simulink model "Controller_Exp"  (R2016a)
settings: Solver=ode4  StartTime=0.0  StopTime=Inf  FixedStep=Ts  RelTol=1e-3
undefined symbols (not defined in the file or in its folder): A_lpf_velocity, B1_lpf_velocity, B2_lpf_velocity, Calibration, commanded_u, GearOffsets, IMUTorsoOffsets, MedullaCommand, ResetDAQ, sample_time, TorsoCOMOffsets, Ts
libraries: xpcethercatlib x188, simulink x37, slrtlib x11, ControllerLibrary x2, dspswit3 x1
(part 3 of 4)

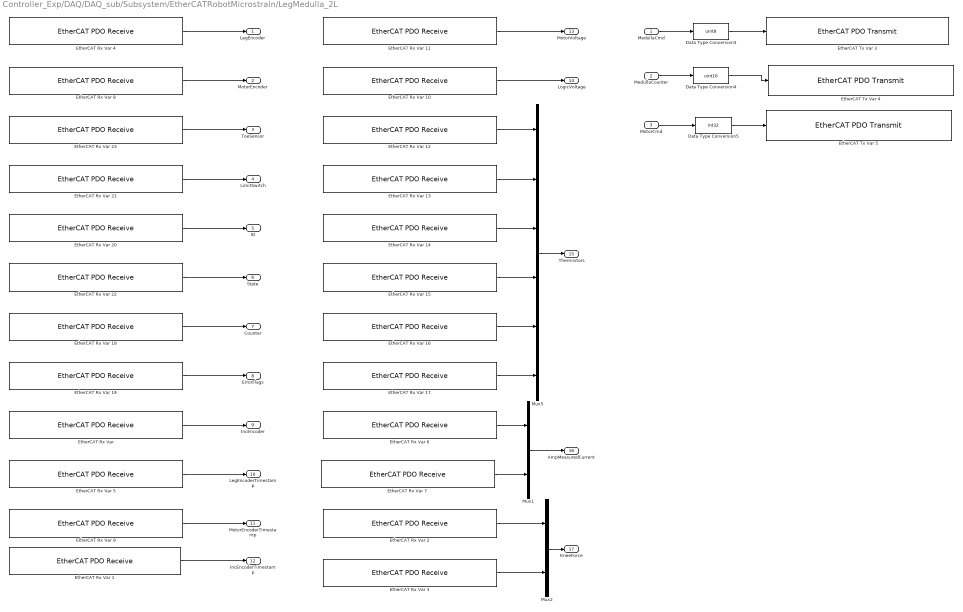
== system Controller_Exp/DAQ/DAQ_sub/Subsystem/EtherCATRobotMicrostrain/LegMedulla_2L ==
  MedullaCmd : Inport
  MedullaCounter : Inport  Port=2
  MotorCmd : Inport  Port=3
  Data Type Conversion3 : DataTypeConversion  OutDataTypeStr=uint8  RndMeth=Simplest
  Data Type Conversion4 : DataTypeConversion  OutDataTypeStr=uint16  RndMeth=Simplest
  Data Type Conversion5 : DataTypeConversion  OutDataTypeStr=int32  RndMeth=Simplest
  "EtherCAT Rx Var " : xpcethercatlib/EtherCAT PDO Receive  Priority=2  sig_name=Box 6 (ATRIAS 2.1 Leg (Medulla 1.5)).Incremental Encoder.Incremental Encoder  sig_offset=1624  sig_type=uint16  type_size=16  sig_dim=1  device_id=3  sample_time=0.001000
  EtherCAT Rx Var 1 : xpcethercatlib/EtherCAT PDO Receive  Priority=2  sig_name=Box 6 (ATRIAS 2.1 Leg (Medulla 1.5)).Incremental Encoder.Incremental Encoder Timestamp  sig_offset=1640  sig_type=uint16  type_size=16  sig_dim=1  device_id=3  sample_time=0.001000
  EtherCAT Rx Var 10 : xpcethercatlib/EtherCAT PDO Receive  Priority=2  sig_name=Box 6 (ATRIAS 2.1 Leg (Medulla 1.5)).Power.Logic Voltage  sig_offset=1672  sig_type=uint16  type_size=16  sig_dim=1  device_id=3  sample_time=0.001000
  EtherCAT Rx Var 11 : xpcethercatlib/EtherCAT PDO Receive  Priority=2  sig_name=Box 6 (ATRIAS 2.1 Leg (Medulla 1.5)).Power.Motor Voltage  sig_offset=1656  sig_type=uint16  type_size=16  sig_dim=1  device_id=3  sample_time=0.001000
  EtherCAT Rx Var 12 : xpcethercatlib/EtherCAT PDO Receive  Priority=2  sig_name=Box 6 (ATRIAS 2.1 Leg (Medulla 1.5)).Thermistors.Thermistor 0  sig_offset=1688  sig_type=uint16  type_size=16  sig_dim=1  device_id=3  sample_time=0.001000
  EtherCAT Rx Var 13 : xpcethercatlib/EtherCAT PDO Receive  Priority=2  sig_name=Box 6 (ATRIAS 2.1 Leg (Medulla 1.5)).Thermistors.Thermistor 1  sig_offset=1704  sig_type=uint16  type_size=16  sig_dim=1  device_id=3  sample_time=0.001000
  EtherCAT Rx Var 14 : xpcethercatlib/EtherCAT PDO Receive  Priority=2  sig_name=Box 6 (ATRIAS 2.1 Leg (Medulla 1.5)).Thermistors.Thermistor 2  sig_offset=1720  sig_type=uint16  type_size=16  sig_dim=1  device_id=3  sample_time=0.001000
  EtherCAT Rx Var 15 : xpcethercatlib/EtherCAT PDO Receive  Priority=2  sig_name=Box 6 (ATRIAS 2.1 Leg (Medulla 1.5)).Thermistors.Thermistor 3  sig_offset=1736  sig_type=uint16  type_size=16  sig_dim=1  device_id=3  sample_time=0.001000
  EtherCAT Rx Var 16 : xpcethercatlib/EtherCAT PDO Receive  Priority=2  sig_name=Box 6 (ATRIAS 2.1 Leg (Medulla 1.5)).Thermistors.Thermistor 4  sig_offset=1752  sig_type=uint16  type_size=16  sig_dim=1  device_id=3  sample_time=0.001000
  EtherCAT Rx Var 17 : xpcethercatlib/EtherCAT PDO Receive  Priority=2  sig_name=Box 6 (ATRIAS 2.1 Leg (Medulla 1.5)).Thermistors.Thermistor 5  sig_offset=1768  sig_type=uint16  type_size=16  sig_dim=1  device_id=3  sample_time=0.001000
  EtherCAT Rx Var 18 : xpcethercatlib/EtherCAT PDO Receive  Priority=2  sig_name=Box 6 (ATRIAS 2.1 Leg (Medulla 1.5)).uController Status.Counter  sig_offset=1488  sig_type=uint8  type_size=8  sig_dim=1  device_id=3  sample_time=0.001000
  EtherCAT Rx Var 19 : xpcethercatlib/EtherCAT PDO Receive  Priority=2  sig_name=Box 6 (ATRIAS 2.1 Leg (Medulla 1.5)).uController Status.Error Flags  sig_offset=1496  sig_type=uint8  type_size=8  sig_dim=1  device_id=3  sample_time=0.001000
  EtherCAT Rx Var 2 : xpcethercatlib/EtherCAT PDO Receive  Priority=2  sig_name=Box 6 (ATRIAS 2.1 Leg (Medulla 1.5)).Knee Force.Knee Force 1  sig_offset=1816  sig_type=uint16  type_size=16  sig_dim=1  device_id=3  sample_time=0.001000
  EtherCAT Rx Var 20 : xpcethercatlib/EtherCAT PDO Receive  Priority=2  sig_name=Box 6 (ATRIAS 2.1 Leg (Medulla 1.5)).uController Status.ID  sig_offset=1472  sig_type=uint8  type_size=8  sig_dim=1  device_id=3  sample_time=0.001000
  EtherCAT Rx Var 21 : xpcethercatlib/EtherCAT PDO Receive  Priority=2  sig_name=Box 6 (ATRIAS 2.1 Leg (Medulla 1.5)).uController Status.Limit Switch  sig_offset=1504  sig_type=uint8  type_size=8  sig_dim=1  device_id=3  sample_time=0.001000
  EtherCAT Rx Var 22 : xpcethercatlib/EtherCAT PDO Receive  Priority=2  sig_name=Box 6 (ATRIAS 2.1 Leg (Medulla 1.5)).uController Status.State  sig_offset=1480  sig_type=uint8  type_size=8  sig_dim=1  device_id=3  sample_time=0.001000
  EtherCAT Rx Var 23 : xpcethercatlib/EtherCAT PDO Receive  Priority=2  sig_name=Box 6 (ATRIAS 2.1 Leg (Medulla 1.5)).uController Status.Toe Sensor  sig_offset=1512  sig_type=uint16  type_size=16  sig_dim=1  device_id=3  sample_time=0.001000
  EtherCAT Rx Var 3 : xpcethercatlib/EtherCAT PDO Receive  Priority=2  sig_name=Box 6 (ATRIAS 2.1 Leg (Medulla 1.5)).Knee Force.Knee Force 2  sig_offset=1832  sig_type=uint16  type_size=16  sig_dim=1  device_id=3  sample_time=0.001000
  EtherCAT Rx Var 4 : xpcethercatlib/EtherCAT PDO Receive  Priority=2  sig_name=Box 6 (ATRIAS 2.1 Leg (Medulla 1.5)).Leg Encoder.Leg Encoder  sig_offset=1576  sig_type=uint32  type_size=32  sig_dim=1  device_id=3  sample_time=0.001000
  EtherCAT Rx Var 5 : xpcethercatlib/EtherCAT PDO Receive  Priority=2  sig_name=Box 6 (ATRIAS 2.1 Leg (Medulla 1.5)).Leg Encoder.Leg Encoder Timestamp  sig_offset=1608  sig_type=uint16  type_size=16  sig_dim=1  device_id=3  sample_time=0.001000
  EtherCAT Rx Var 6 : xpcethercatlib/EtherCAT PDO Receive  Priority=2  sig_name=Box 6 (ATRIAS 2.1 Leg (Medulla 1.5)).Measured Current.Amp 1 Measured Current  sig_offset=1784  sig_type=int16  type_size=16  sig_dim=1  device_id=3  sample_time=0.001000
  EtherCAT Rx Var 7 : xpcethercatlib/EtherCAT PDO Receive  Priority=2  sig_name=Box 6 (ATRIAS 2.1 Leg (Medulla 1.5)).Measured Current.Amp 2 Measured Current  sig_offset=1800  sig_type=int16  type_size=16  sig_dim=1  device_id=3  sample_time=0.001000
  EtherCAT Rx Var 8 : xpcethercatlib/EtherCAT PDO Receive  Priority=2  sig_name=Box 6 (ATRIAS 2.1 Leg (Medulla 1.5)).Motor Encoder.Motor Encoder  sig_offset=1528  sig_type=uint32  type_size=32  sig_dim=1  device_id=3  sample_time=0.001000
  EtherCAT Rx Var 9 : xpcethercatlib/EtherCAT PDO Receive  Priority=2  sig_name=Box 6 (ATRIAS 2.1 Leg (Medulla 1.5)).Motor Encoder.Motor Encoder Timestamp  sig_offset=1560  sig_type=uint16  type_size=16  sig_dim=1  device_id=3  sample_time=0.001000
  EtherCAT Tx Var 3 : xpcethercatlib/EtherCAT PDO Transmit   Priority=3  sig_name=Box 6 (ATRIAS 2.1 Leg (Medulla 1.5)).uControllerInput.Command  sig_offset=1472  sig_type=uint8  type_size=8  sig_dim=1  device_id=3  sample_time=0.001000
  EtherCAT Tx Var 4 : xpcethercatlib/EtherCAT PDO Transmit   Priority=3  sig_name=Box 6 (ATRIAS 2.1 Leg (Medulla 1.5)).uControllerInput.Counter  sig_offset=1480  sig_type=uint16  type_size=16  sig_dim=1  device_id=3  sample_time=0.001000
  EtherCAT Tx Var 5 : xpcethercatlib/EtherCAT PDO Transmit   Priority=3  sig_name=Box 6 (ATRIAS 2.1 Leg (Medulla 1.5)).uControllerInput.Motor Current  sig_offset=1496  sig_type=int32  type_size=32  sig_dim=1  device_id=3  sample_time=0.001000
  Mux1 : Mux  Inputs=2
  Mux2 : Mux  Inputs=2
  Mux5 : Mux  Inputs=6
  LegEncoder : Outport
  MotorEncoder : Outport  Port=2
  ToeSensor : Outport  Port=3
  LimitSwitch : Outport  Port=4
  ID : Outport  Port=5
  State : Outport  Port=6
  Counter : Outport  Port=7
  ErrorFlags : Outport  Port=8
  IncEncoder : Outport  Port=9
  LegEncoderTimestamp : Outport  Port=10
  MotorEncoderTimestamp : Outport  Port=11
  IncEncoderTimestamp : Outport  Port=12
  MotorVoltage : Outport  Port=13
  LogicVoltage : Outport  Port=14
  Thermistors : Outport  Port=15
  AmpMeasuredCurrent : Outport  Port=16
  KneeForce : Outport  Port=17
  wires:
  Mux2/1 -> KneeForce/1
  Mux1/1 -> AmpMeasuredCurrent/1
  Mux5/1 -> Thermistors/1
  MotorCmd/1 -> Data Type Conversion5/1
  MedullaCounter/1 -> Data Type Conversion4/1
  MedullaCmd/1 -> Data Type Conversion3/1
  EtherCAT Rx Var 23/1 -> ToeSensor/1
  EtherCAT Rx Var 22/1 -> State/1
  EtherCAT Rx Var 21/1 -> LimitSwitch/1
  EtherCAT Rx Var 20/1 -> ID/1
  EtherCAT Rx Var 19/1 -> ErrorFlags/1
  EtherCAT Rx Var 18/1 -> Counter/1
  EtherCAT Rx Var 17/1 -> Mux5/6
  EtherCAT Rx Var 16/1 -> Mux5/5
  EtherCAT Rx Var 15/1 -> Mux5/4
  EtherCAT Rx Var 14/1 -> Mux5/3
  EtherCAT Rx Var 13/1 -> Mux5/2
  EtherCAT Rx Var 12/1 -> Mux5/1
  EtherCAT Rx Var 11/1 -> MotorVoltage/1
  EtherCAT Rx Var 10/1 -> LogicVoltage/1
  EtherCAT Rx Var 9/1 -> MotorEncoderTimestamp/1
  EtherCAT Rx Var 8/1 -> MotorEncoder/1
  EtherCAT Rx Var 7/1 -> Mux1/2
  EtherCAT Rx Var 6/1 -> Mux1/1
  EtherCAT Rx Var 5/1 -> LegEncoderTimestamp/1
  EtherCAT Rx Var 4/1 -> LegEncoder/1
  EtherCAT Rx Var 3/1 -> Mux2/2
  EtherCAT Rx Var 2/1 -> Mux2/1
  EtherCAT Rx Var 1/1 -> IncEncoderTimestamp/1
  "EtherCAT Rx Var "/1 -> IncEncoder/1
  Data Type Conversion5/1 -> EtherCAT Tx Var 5/1
  Data Type Conversion4/1 -> EtherCAT Tx Var 4/1
  Data Type Conversion3/1 -> EtherCAT Tx Var 3/1

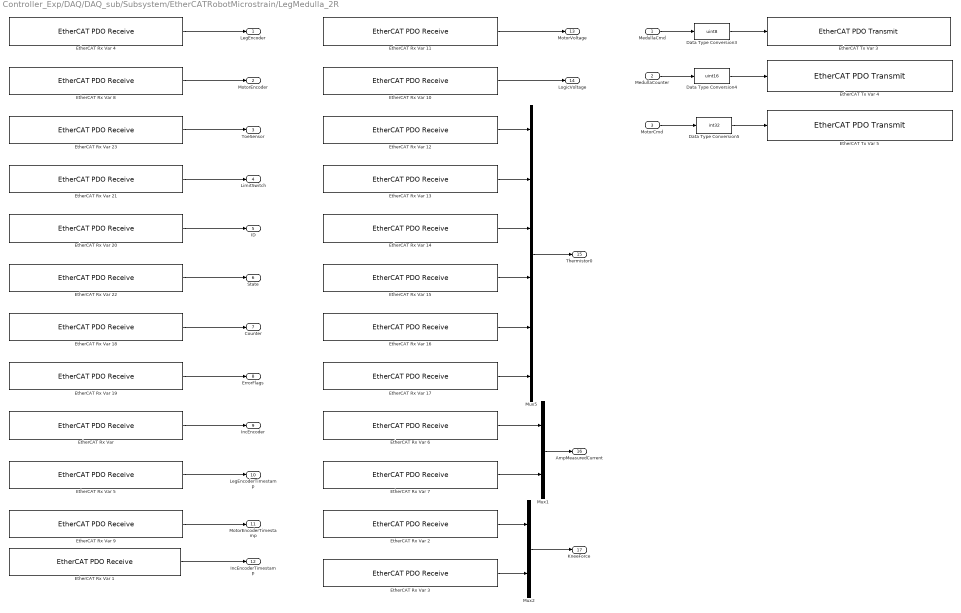
== system Controller_Exp/DAQ/DAQ_sub/Subsystem/EtherCATRobotMicrostrain/LegMedulla_2R ==
  MedullaCmd : Inport
  MedullaCounter : Inport  Port=2
  MotorCmd : Inport  Port=3
  Data Type Conversion3 : DataTypeConversion  OutDataTypeStr=uint8  RndMeth=Simplest
  Data Type Conversion4 : DataTypeConversion  OutDataTypeStr=uint16  RndMeth=Simplest
  Data Type Conversion5 : DataTypeConversion  OutDataTypeStr=int32  RndMeth=Simplest
  "EtherCAT Rx Var " : xpcethercatlib/EtherCAT PDO Receive  Priority=2  sig_name=Box 7 (ATRIAS 2.1 Leg (Medulla 1.5)).Incremental Encoder.Incremental Encoder  sig_offset=2000  sig_type=uint16  type_size=16  sig_dim=1  device_id=3  sample_time=0.001000
  EtherCAT Rx Var 1 : xpcethercatlib/EtherCAT PDO Receive  Priority=2  sig_name=Box 7 (ATRIAS 2.1 Leg (Medulla 1.5)).Incremental Encoder.Incremental Encoder Timestamp  sig_offset=2016  sig_type=uint16  type_size=16  sig_dim=1  device_id=3  sample_time=0.001000
  EtherCAT Rx Var 10 : xpcethercatlib/EtherCAT PDO Receive  Priority=2  sig_name=Box 7 (ATRIAS 2.1 Leg (Medulla 1.5)).Power.Logic Voltage  sig_offset=2048  sig_type=uint16  type_size=16  sig_dim=1  device_id=3  sample_time=0.001000
  EtherCAT Rx Var 11 : xpcethercatlib/EtherCAT PDO Receive  Priority=2  sig_name=Box 7 (ATRIAS 2.1 Leg (Medulla 1.5)).Power.Motor Voltage  sig_offset=2032  sig_type=uint16  type_size=16  sig_dim=1  device_id=3  sample_time=0.001000
  EtherCAT Rx Var 12 : xpcethercatlib/EtherCAT PDO Receive  Priority=2  sig_name=Box 7 (ATRIAS 2.1 Leg (Medulla 1.5)).Thermistors.Thermistor 0  sig_offset=2064  sig_type=uint16  type_size=16  sig_dim=1  device_id=3  sample_time=0.001000
  EtherCAT Rx Var 13 : xpcethercatlib/EtherCAT PDO Receive  Priority=2  sig_name=Box 7 (ATRIAS 2.1 Leg (Medulla 1.5)).Thermistors.Thermistor 1  sig_offset=2080  sig_type=uint16  type_size=16  sig_dim=1  device_id=3  sample_time=0.001000
  EtherCAT Rx Var 14 : xpcethercatlib/EtherCAT PDO Receive  Priority=2  sig_name=Box 7 (ATRIAS 2.1 Leg (Medulla 1.5)).Thermistors.Thermistor 2  sig_offset=2096  sig_type=uint16  type_size=16  sig_dim=1  device_id=3  sample_time=0.001000
  EtherCAT Rx Var 15 : xpcethercatlib/EtherCAT PDO Receive  Priority=2  sig_name=Box 7 (ATRIAS 2.1 Leg (Medulla 1.5)).Thermistors.Thermistor 3  sig_offset=2112  sig_type=uint16  type_size=16  sig_dim=1  device_id=3  sample_time=0.001000
  EtherCAT Rx Var 16 : xpcethercatlib/EtherCAT PDO Receive  Priority=2  sig_name=Box 7 (ATRIAS 2.1 Leg (Medulla 1.5)).Thermistors.Thermistor 4  sig_offset=2128  sig_type=uint16  type_size=16  sig_dim=1  device_id=3  sample_time=0.001000
  EtherCAT Rx Var 17 : xpcethercatlib/EtherCAT PDO Receive  Priority=2  sig_name=Box 7 (ATRIAS 2.1 Leg (Medulla 1.5)).Thermistors.Thermistor 5  sig_offset=2144  sig_type=uint16  type_size=16  sig_dim=1  device_id=3  sample_time=0.001000
  EtherCAT Rx Var 18 : xpcethercatlib/EtherCAT PDO Receive  Priority=2  sig_name=Box 7 (ATRIAS 2.1 Leg (Medulla 1.5)).uController Status.Counter  sig_offset=1864  sig_type=uint8  type_size=8  sig_dim=1  device_id=3  sample_time=0.001000
  EtherCAT Rx Var 19 : xpcethercatlib/EtherCAT PDO Receive  Priority=2  sig_name=Box 7 (ATRIAS 2.1 Leg (Medulla 1.5)).uController Status.Error Flags  sig_offset=1872  sig_type=uint8  type_size=8  sig_dim=1  device_id=3  sample_time=0.001000
  EtherCAT Rx Var 2 : xpcethercatlib/EtherCAT PDO Receive  Priority=2  sig_name=Box 7 (ATRIAS 2.1 Leg (Medulla 1.5)).Knee Force.Knee Force 1  sig_offset=2192  sig_type=uint16  type_size=16  sig_dim=1  device_id=3  sample_time=0.001000
  EtherCAT Rx Var 20 : xpcethercatlib/EtherCAT PDO Receive  Priority=2  sig_name=Box 7 (ATRIAS 2.1 Leg (Medulla 1.5)).uController Status.ID  sig_offset=1848  sig_type=uint8  type_size=8  sig_dim=1  device_id=3  sample_time=0.001000
  EtherCAT Rx Var 21 : xpcethercatlib/EtherCAT PDO Receive  Priority=2  sig_name=Box 7 (ATRIAS 2.1 Leg (Medulla 1.5)).uController Status.Limit Switch  sig_offset=1880  sig_type=uint8  type_size=8  sig_dim=1  device_id=3  sample_time=0.001000
  EtherCAT Rx Var 22 : xpcethercatlib/EtherCAT PDO Receive  Priority=2  sig_name=Box 7 (ATRIAS 2.1 Leg (Medulla 1.5)).uController Status.State  sig_offset=1856  sig_type=uint8  type_size=8  sig_dim=1  device_id=3  sample_time=0.001000
  EtherCAT Rx Var 23 : xpcethercatlib/EtherCAT PDO Receive  Priority=2  sig_name=Box 7 (ATRIAS 2.1 Leg (Medulla 1.5)).uController Status.Toe Sensor  sig_offset=1888  sig_type=uint16  type_size=16  sig_dim=1  device_id=3  sample_time=0.001000
  EtherCAT Rx Var 3 : xpcethercatlib/EtherCAT PDO Receive  Priority=2  sig_name=Box 7 (ATRIAS 2.1 Leg (Medulla 1.5)).Knee Force.Knee Force 2  sig_offset=2208  sig_type=uint16  type_size=16  sig_dim=1  device_id=3  sample_time=0.001000
  EtherCAT Rx Var 4 : xpcethercatlib/EtherCAT PDO Receive  Priority=2  sig_name=Box 7 (ATRIAS 2.1 Leg (Medulla 1.5)).Leg Encoder.Leg Encoder  sig_offset=1952  sig_type=uint32  type_size=32  sig_dim=1  device_id=3  sample_time=0.001000
  EtherCAT Rx Var 5 : xpcethercatlib/EtherCAT PDO Receive  Priority=2  sig_name=Box 7 (ATRIAS 2.1 Leg (Medulla 1.5)).Leg Encoder.Leg Encoder Timestamp  sig_offset=1984  sig_type=uint16  type_size=16  sig_dim=1  device_id=3  sample_time=0.001000
  EtherCAT Rx Var 6 : xpcethercatlib/EtherCAT PDO Receive  Priority=2  sig_name=Box 7 (ATRIAS 2.1 Leg (Medulla 1.5)).Measured Current.Amp 1 Measured Current  sig_offset=2160  sig_type=int16  type_size=16  sig_dim=1  device_id=3  sample_time=0.001000
  EtherCAT Rx Var 7 : xpcethercatlib/EtherCAT PDO Receive  Priority=2  sig_name=Box 7 (ATRIAS 2.1 Leg (Medulla 1.5)).Measured Current.Amp 2 Measured Current  sig_offset=2176  sig_type=int16  type_size=16  sig_dim=1  device_id=3  sample_time=0.001000
  EtherCAT Rx Var 8 : xpcethercatlib/EtherCAT PDO Receive  Priority=2  sig_name=Box 7 (ATRIAS 2.1 Leg (Medulla 1.5)).Motor Encoder.Motor Encoder  sig_offset=1904  sig_type=uint32  type_size=32  sig_dim=1  device_id=3  sample_time=0.001000
  EtherCAT Rx Var 9 : xpcethercatlib/EtherCAT PDO Receive  Priority=2  sig_name=Box 7 (ATRIAS 2.1 Leg (Medulla 1.5)).Motor Encoder.Motor Encoder Timestamp  sig_offset=1936  sig_type=uint16  type_size=16  sig_dim=1  device_id=3  sample_time=0.001000
  EtherCAT Tx Var 3 : xpcethercatlib/EtherCAT PDO Transmit   Priority=3  sig_name=Box 7 (ATRIAS 2.1 Leg (Medulla 1.5)).uControllerInput.Command  sig_offset=1848  sig_type=uint8  type_size=8  sig_dim=1  device_id=3  sample_time=0.001000
  EtherCAT Tx Var 4 : xpcethercatlib/EtherCAT PDO Transmit   Priority=3  sig_name=Box 7 (ATRIAS 2.1 Leg (Medulla 1.5)).uControllerInput.Counter  sig_offset=1856  sig_type=uint16  type_size=16  sig_dim=1  device_id=3  sample_time=0.001000
  EtherCAT Tx Var 5 : xpcethercatlib/EtherCAT PDO Transmit   Priority=3  sig_name=Box 7 (ATRIAS 2.1 Leg (Medulla 1.5)).uControllerInput.Motor Current  sig_offset=1872  sig_type=int32  type_size=32  sig_dim=1  device_id=3  sample_time=0.001000
  Mux1 : Mux  Inputs=2
  Mux2 : Mux  Inputs=2
  Mux5 : Mux  Inputs=6
  LegEncoder : Outport
  MotorEncoder : Outport  Port=2
  ToeSensor : Outport  Port=3
  LimitSwitch : Outport  Port=4
  ID : Outport  Port=5
  State : Outport  Port=6
  Counter : Outport  Port=7
  ErrorFlags : Outport  Port=8
  IncEncoder : Outport  Port=9
  LegEncoderTimestamp : Outport  Port=10
  MotorEncoderTimestamp : Outport  Port=11
  IncEncoderTimestamp : Outport  Port=12
  MotorVoltage : Outport  Port=13
  LogicVoltage : Outport  Port=14
  Thermistor0 : Outport  Port=15
  AmpMeasuredCurrent : Outport  Port=16
  KneeForce : Outport  Port=17
  wires:
  Mux2/1 -> KneeForce/1
  Mux1/1 -> AmpMeasuredCurrent/1
  Mux5/1 -> Thermistor0/1
  MotorCmd/1 -> Data Type Conversion5/1
  MedullaCounter/1 -> Data Type Conversion4/1
  MedullaCmd/1 -> Data Type Conversion3/1
  EtherCAT Rx Var 23/1 -> ToeSensor/1
  EtherCAT Rx Var 22/1 -> State/1
  EtherCAT Rx Var 21/1 -> LimitSwitch/1
  EtherCAT Rx Var 20/1 -> ID/1
  EtherCAT Rx Var 19/1 -> ErrorFlags/1
  EtherCAT Rx Var 18/1 -> Counter/1
  EtherCAT Rx Var 17/1 -> Mux5/6
  EtherCAT Rx Var 16/1 -> Mux5/5
  EtherCAT Rx Var 15/1 -> Mux5/4
  EtherCAT Rx Var 14/1 -> Mux5/3
  EtherCAT Rx Var 13/1 -> Mux5/2
  EtherCAT Rx Var 12/1 -> Mux5/1
  EtherCAT Rx Var 11/1 -> MotorVoltage/1
  EtherCAT Rx Var 10/1 -> LogicVoltage/1
  EtherCAT Rx Var 9/1 -> MotorEncoderTimestamp/1
  EtherCAT Rx Var 8/1 -> MotorEncoder/1
  EtherCAT Rx Var 7/1 -> Mux1/2
  EtherCAT Rx Var 6/1 -> Mux1/1
  EtherCAT Rx Var 5/1 -> LegEncoderTimestamp/1
  EtherCAT Rx Var 4/1 -> LegEncoder/1
  EtherCAT Rx Var 3/1 -> Mux2/2
  EtherCAT Rx Var 2/1 -> Mux2/1
  EtherCAT Rx Var 1/1 -> IncEncoderTimestamp/1
  "EtherCAT Rx Var "/1 -> IncEncoder/1
  Data Type Conversion5/1 -> EtherCAT Tx Var 5/1
  Data Type Conversion4/1 -> EtherCAT Tx Var 4/1
  Data Type Conversion3/1 -> EtherCAT Tx Var 3/1

== system Controller_Exp/DAQ/DAQ_sub/Subsystem/EncoderFilters/Filter/Velocity Filter ==
  q : Inport
  Delay : Delay  DelayLength=1
  Delay1 : Delay
  Delay2 : Delay  DelayLength=3
  Delay3 : Delay  DelayLength=4
  Delay4 : Delay  DelayLength=5
  Delay5 : Delay  DelayLength=6
  Delay6 : Delay  DelayLength=7
  Delay7 : Delay  DelayLength=8
  Delay8 : Delay  DelayLength=9
  Median Filter : MATLAB Function  TreatAsAtomicUnit=on
  OSU_filter : Subsystem
  Vector Concatenate : Concatenate  NumInputs=9  Mode=Multidimensional array  ConcatenateDimension=2
  dq_out : Outport
  dq_original : Outport  Port=2
  wires:
  Median Filter/1(dq_out) -> dq_out/1
  q/1 -> OSU_filter/1(q)
  Vector Concatenate/1 -> Median Filter/2(dq_past)
  Delay/1 -> Vector Concatenate/1
  Delay1/1 -> Vector Concatenate/2
  Delay2/1 -> Vector Concatenate/3
  Delay3/1 -> Vector Concatenate/4
  Delay4/1 -> Vector Concatenate/5
  Delay5/1 -> Vector Concatenate/6
  Delay6/1 -> Vector Concatenate/7
  Delay7/1 -> Vector Concatenate/8
  Delay8/1 -> Vector Concatenate/9
  OSU_filter/1(dq) -> Median Filter/1(dq), Delay8/1, Delay7/1, Delay6/1, Delay5/1, Delay4/1, Delay3/1, Delay2/1, Delay1/1, Delay/1, dq_original/1

== system Controller_Exp/DAQ/DAQ_sub/Subsystem/EncoderFilters1/CheckAndFilterEncoder/Velocity Filter ==
  In1 : Inport
  Logic Filter : MATLAB Function  TreatAsAtomicUnit=on
  OSU_filter : Subsystem
  Unit Delay1 : UnitDelay  SampleTime=-1
  Unit Delay2 : UnitDelay  SampleTime=-1
  Out1 : Outport
  Out2 : Outport  Port=2
  wires:
  Logic Filter/1(dq_out) -> Out1/1
  OSU_filter/1(dq) -> Logic Filter/1(dq), Unit Delay2/1, Out2/1
  In1/1 -> OSU_filter/1(q)
  Unit Delay2/1 -> Logic Filter/2(dq_prev)
  Logic Filter/2(dq_good) -> Unit Delay1/1
  Unit Delay1/1 -> Logic Filter/3(dq_good_prev)

== system Controller_Exp/DAQ/DAQ_sub/Subsystem/EtherCATRobotMicrostrain/LegElmo_1L/EtherCATSubsystem ==
  TargetTorque : Inport
  ControlWord : Inport  Port=2
  ModeOfOperation : Inport  Port=3
  EtherCAT PDO Receive : xpcethercatlib/EtherCAT PDO Receive  Priority=2  sig_name=Box 3 (Elmo Drive).Inputs.Torque actual value  sig_offset=3024  sig_type=int16  type_size=16  sig_dim=1  device_id=3  sample_time=0.001000
  EtherCAT PDO Receive1 : xpcethercatlib/EtherCAT PDO Receive  Priority=2  sig_name=Box 3 (Elmo Drive).Inputs.Position actual value  sig_offset=2992  sig_type=int32  type_size=32  sig_dim=1  device_id=3  sample_time=0.001000
  EtherCAT PDO Receive2 : xpcethercatlib/EtherCAT PDO Receive  Priority=2  sig_name=Box 3 (Elmo Drive).Inputs.Mode of operation display  sig_offset=3056  sig_type=int8  type_size=8  sig_dim=1  device_id=3  sample_time=0.001000
  EtherCAT PDO Receive5 : xpcethercatlib/EtherCAT PDO Receive  Priority=2  sig_name=Box 3 (Elmo Drive).Inputs.Status word  sig_offset=3040  sig_type=uint16  type_size=16  sig_dim=1  device_id=3  sample_time=0.001000
  EtherCAT PDO Transmit : xpcethercatlib/EtherCAT PDO Transmit   Priority=3  sig_name=Box 3 (Elmo Drive).Outputs.Target Torque  sig_offset=2992  sig_type=int16  type_size=16  sig_dim=1  device_id=3  sample_time=0.001000
  EtherCAT PDO Transmit1 : xpcethercatlib/EtherCAT PDO Transmit   Priority=3  sig_name=Box 3 (Elmo Drive).Outputs.Control word  sig_offset=3008  sig_type=uint16  type_size=16  sig_dim=1  device_id=3  sample_time=0.001000
  EtherCAT PDO Transmit2 : xpcethercatlib/EtherCAT PDO Transmit   Priority=3  sig_name=Box 3 (Elmo Drive).Outputs.Mode of operation  sig_offset=3024  sig_type=int8  type_size=8  sig_dim=1  device_id=3  sample_time=0.001000
  TorqueActual : Outport
  ActualPosition : Outport  Port=2
  ModeOfOperationDisplay : Outport  Port=3
  StatusWord : Outport  Port=4
  wires:
  EtherCAT PDO Receive5/1 -> StatusWord/1
  TargetTorque/1 -> EtherCAT PDO Transmit/1
  EtherCAT PDO Receive2/1 -> ModeOfOperationDisplay/1
  ModeOfOperation/1 -> EtherCAT PDO Transmit2/1
  ControlWord/1 -> EtherCAT PDO Transmit1/1
  EtherCAT PDO Receive1/1 -> ActualPosition/1
  EtherCAT PDO Receive/1 -> TorqueActual/1

== system Controller_Exp/DAQ/DAQ_sub/Subsystem/EtherCATRobotMicrostrain/LegElmo_1L/Subsystem ==
  ActualValue : Inport
  MaxRatedCurrent : Inport  Port=2
  Data Type Conversion6 : DataTypeConversion  OutDataTypeStr=int16
  Fcn : Fcn  Expr=u(1)*1000/u(2)
  Vector Concatenate : Concatenate
  ScaledValue : Outport
  wires:
  Fcn/1 -> Data Type Conversion6/1
  Data Type Conversion6/1 -> ScaledValue/1
  MaxRatedCurrent/1 -> Vector Concatenate/2
  Vector Concatenate/1 -> Fcn/1
  ActualValue/1 -> Vector Concatenate/1

== system Controller_Exp/DAQ/DAQ_sub/Subsystem/EtherCATRobotMicrostrain/LegElmo_1L/Subsystem1 ==
  ControlWordIndex : Inport
  EnableControlWord : Subsystem
  FaultReset : Subsystem
  Merge : Merge  Inputs=4
  NothingControlWord : Subsystem
  ShutdownControlWord : Subsystem
  Switch Case : SwitchCase  CaseConditions={1,2,3}
  ControlWord : Outport
  wires:
  FaultReset/1(ControlWord) -> Merge/3
  Switch Case/3 -> FaultReset/Action
  EnableControlWord/1(ControlWord) -> Merge/2
  ControlWordIndex/1 -> Switch Case/1
  Switch Case/2 -> EnableControlWord/Action
  Switch Case/4 -> NothingControlWord/Action
  ShutdownControlWord/1(ControlWord) -> Merge/1
  Switch Case/1 -> ShutdownControlWord/Action
  Merge/1 -> ControlWord/1
  NothingControlWord/1(ControlWord) -> Merge/4

== system Controller_Exp/DAQ/DAQ_sub/Subsystem/EtherCATRobotMicrostrain/LegElmo_1L/Subsystem2 ==
  StatusWord : Inport
  Bitwise Operator : simulink/Logic and Bit Operations/Bitwise Operator  logicop=AND  UseBitMask=on  BitMask=bin2dec('0000000001001111')  BitMaskRealWorld=Stored Integer
  Compare To Constant : simulink/Logic and Bit Operations/Compare To Constant  relop===  const=bin2dec('0000000001000000')  OutDataTypeStr=boolean
  SwitchOnDisabledMode : Outport
  wires:
  Bitwise Operator/1 -> Compare To Constant/1
  Compare To Constant/1 -> SwitchOnDisabledMode/1
  StatusWord/1 -> Bitwise Operator/1

== system Controller_Exp/DAQ/DAQ_sub/Subsystem/EtherCATRobotMicrostrain/LegElmo_1L/Subsystem3 ==
  StatusWord : Inport
  Bitwise Operator : simulink/Logic and Bit Operations/Bitwise Operator  logicop=AND  UseBitMask=on  BitMask=bin2dec('0000000001101111')  BitMaskRealWorld=Stored Integer
  Compare To Constant : simulink/Logic and Bit Operations/Compare To Constant  relop===  const=bin2dec('0000000000100111')  OutDataTypeStr=boolean
  EnabledMode : Outport
  wires:
  Bitwise Operator/1 -> Compare To Constant/1
  Compare To Constant/1 -> EnabledMode/1
  StatusWord/1 -> Bitwise Operator/1

== system Controller_Exp/DAQ/DAQ_sub/Subsystem/EtherCATRobotMicrostrain/LegElmo_1L/Subsystem4 ==
  StatusWord : Inport
  Bitwise Operator : simulink/Logic and Bit Operations/Bitwise Operator  logicop=AND  UseBitMask=on  BitMask=bin2dec('0000000001101111')  BitMaskRealWorld=Stored Integer
  Compare To Constant : simulink/Logic and Bit Operations/Compare To Constant  relop===  const=bin2dec('0000000000100001')  OutDataTypeStr=boolean
  ReadyToSwitchOnMode : Outport
  wires:
  Bitwise Operator/1 -> Compare To Constant/1
  Compare To Constant/1 -> ReadyToSwitchOnMode/1
  StatusWord/1 -> Bitwise Operator/1

== system Controller_Exp/DAQ/DAQ_sub/Subsystem/EtherCATRobotMicrostrain/LegElmo_1L/Subsystem5 ==
  StatusWord : Inport
  Bitwise Operator : simulink/Logic and Bit Operations/Bitwise Operator  logicop=AND  UseBitMask=on  BitMask=bin2dec('0000000000001000')  BitMaskRealWorld=Stored Integer
  Compare To Constant : simulink/Logic and Bit Operations/Compare To Constant  relop===  const=bin2dec('0000000000001000')  OutDataTypeStr=boolean
  FaultMode : Outport
  wires:
  Bitwise Operator/1 -> Compare To Constant/1
  Compare To Constant/1 -> FaultMode/1
  StatusWord/1 -> Bitwise Operator/1

== system Controller_Exp/DAQ/DAQ_sub/Subsystem/EtherCATRobotMicrostrain/LegElmo_1L/Subsystem6 ==
  ScaledValue : Inport
  MaxRatedCurrent : Inport  Port=2
  Fcn : Fcn  Expr=u(1)*u(2)/1000
  Vector Concatenate : Concatenate
  ActualValue : Outport
  wires:
  Fcn/1 -> ActualValue/1
  MaxRatedCurrent/1 -> Vector Concatenate/2
  Vector Concatenate/1 -> Fcn/1
  ScaledValue/1 -> Vector Concatenate/1

== system Controller_Exp/DAQ/DAQ_sub/Subsystem/EtherCATRobotMicrostrain/LegElmo_1R/EtherCATSubsystem ==
  TargetTorque : Inport
  ControlWord : Inport  Port=2
  ModeOfOperation : Inport  Port=3
  EtherCAT PDO Receive : xpcethercatlib/EtherCAT PDO Receive  Priority=2  sig_name=Box 10 (Elmo Drive).Inputs.Torque actual value  sig_offset=3184  sig_type=int16  type_size=16  sig_dim=1  device_id=3  sample_time=0.001000
  EtherCAT PDO Receive1 : xpcethercatlib/EtherCAT PDO Receive  Priority=2  sig_name=Box 10 (Elmo Drive).Inputs.Position actual value  sig_offset=3152  sig_type=int32  type_size=32  sig_dim=1  device_id=3  sample_time=0.001000
  EtherCAT PDO Receive2 : xpcethercatlib/EtherCAT PDO Receive  Priority=2  sig_name=Box 10 (Elmo Drive).Inputs.Mode of operation display  sig_offset=3216  sig_type=int8  type_size=8  sig_dim=1  device_id=3  sample_time=0.001000
  EtherCAT PDO Receive5 : xpcethercatlib/EtherCAT PDO Receive  Priority=2  sig_name=Box 10 (Elmo Drive).Inputs.Status word  sig_offset=3200  sig_type=uint16  type_size=16  sig_dim=1  device_id=3  sample_time=0.001000
  EtherCAT PDO Transmit : xpcethercatlib/EtherCAT PDO Transmit   Priority=3  sig_name=Box 10 (Elmo Drive).Outputs.Target Torque  sig_offset=3152  sig_type=int16  type_size=16  sig_dim=1  device_id=3  sample_time=0.001000
  EtherCAT PDO Transmit1 : xpcethercatlib/EtherCAT PDO Transmit   Priority=3  sig_name=Box 10 (Elmo Drive).Outputs.Control word  sig_offset=3168  sig_type=uint16  type_size=16  sig_dim=1  device_id=3  sample_time=0.001000
  EtherCAT PDO Transmit2 : xpcethercatlib/EtherCAT PDO Transmit   Priority=3  sig_name=Box 10 (Elmo Drive).Outputs.Mode of operation  sig_offset=3184  sig_type=int8  type_size=8  sig_dim=1  device_id=3  sample_time=0.001000
  TorqueActual : Outport
  ActualPosition : Outport  Port=2
  ModeOfOperationDisplay : Outport  Port=3
  StatusWord : Outport  Port=4
  wires:
  EtherCAT PDO Receive5/1 -> StatusWord/1
  TargetTorque/1 -> EtherCAT PDO Transmit/1
  EtherCAT PDO Receive2/1 -> ModeOfOperationDisplay/1
  ModeOfOperation/1 -> EtherCAT PDO Transmit2/1
  ControlWord/1 -> EtherCAT PDO Transmit1/1
  EtherCAT PDO Receive1/1 -> ActualPosition/1
  EtherCAT PDO Receive/1 -> TorqueActual/1

== system Controller_Exp/DAQ/DAQ_sub/Subsystem/EtherCATRobotMicrostrain/LegElmo_1R/Subsystem ==
  ActualValue : Inport
  MaxRatedCurrent : Inport  Port=2
  Data Type Conversion6 : DataTypeConversion  OutDataTypeStr=int16
  Fcn : Fcn  Expr=u(1)*1000/u(2)
  Vector Concatenate : Concatenate
  ScaledValue : Outport
  wires:
  Fcn/1 -> Data Type Conversion6/1
  Data Type Conversion6/1 -> ScaledValue/1
  MaxRatedCurrent/1 -> Vector Concatenate/2
  Vector Concatenate/1 -> Fcn/1
  ActualValue/1 -> Vector Concatenate/1

== system Controller_Exp/DAQ/DAQ_sub/Subsystem/EtherCATRobotMicrostrain/LegElmo_1R/Subsystem1 ==
  ControlWordIndex : Inport
  EnableControlWord : Subsystem
  FaultReset : Subsystem
  Merge : Merge  Inputs=4
  NothingControlWord : Subsystem
  ShutdownControlWord : Subsystem
  Switch Case : SwitchCase  CaseConditions={1,2,3}
  ControlWord : Outport
  wires:
  FaultReset/1(ControlWord) -> Merge/3
  Switch Case/3 -> FaultReset/Action
  EnableControlWord/1(ControlWord) -> Merge/2
  ControlWordIndex/1 -> Switch Case/1
  Switch Case/2 -> EnableControlWord/Action
  Switch Case/4 -> NothingControlWord/Action
  ShutdownControlWord/1(ControlWord) -> Merge/1
  Switch Case/1 -> ShutdownControlWord/Action
  Merge/1 -> ControlWord/1
  NothingControlWord/1(ControlWord) -> Merge/4

== system Controller_Exp/DAQ/DAQ_sub/Subsystem/EtherCATRobotMicrostrain/LegElmo_1R/Subsystem2 ==
  StatusWord : Inport
  Bitwise Operator : simulink/Logic and Bit Operations/Bitwise Operator  logicop=AND  UseBitMask=on  BitMask=bin2dec('0000000001001111')  BitMaskRealWorld=Stored Integer
  Compare To Constant : simulink/Logic and Bit Operations/Compare To Constant  relop===  const=bin2dec('0000000001000000')  OutDataTypeStr=boolean
  SwitchOnDisabledMode : Outport
  wires:
  Bitwise Operator/1 -> Compare To Constant/1
  Compare To Constant/1 -> SwitchOnDisabledMode/1
  StatusWord/1 -> Bitwise Operator/1

== system Controller_Exp/DAQ/DAQ_sub/Subsystem/EtherCATRobotMicrostrain/LegElmo_1R/Subsystem3 ==
  StatusWord : Inport
  Bitwise Operator : simulink/Logic and Bit Operations/Bitwise Operator  logicop=AND  UseBitMask=on  BitMask=bin2dec('0000000001101111')  BitMaskRealWorld=Stored Integer
  Compare To Constant : simulink/Logic and Bit Operations/Compare To Constant  relop===  const=bin2dec('0000000000100111')  OutDataTypeStr=boolean
  EnabledMode : Outport
  wires:
  Bitwise Operator/1 -> Compare To Constant/1
  Compare To Constant/1 -> EnabledMode/1
  StatusWord/1 -> Bitwise Operator/1

== system Controller_Exp/DAQ/DAQ_sub/Subsystem/EtherCATRobotMicrostrain/LegElmo_1R/Subsystem4 ==
  StatusWord : Inport
  Bitwise Operator : simulink/Logic and Bit Operations/Bitwise Operator  logicop=AND  UseBitMask=on  BitMask=bin2dec('0000000001101111')  BitMaskRealWorld=Stored Integer
  Compare To Constant : simulink/Logic and Bit Operations/Compare To Constant  relop===  const=bin2dec('0000000000100001')  OutDataTypeStr=boolean
  ReadyToSwitchOnMode : Outport
  wires:
  Bitwise Operator/1 -> Compare To Constant/1
  Compare To Constant/1 -> ReadyToSwitchOnMode/1
  StatusWord/1 -> Bitwise Operator/1

== system Controller_Exp/DAQ/DAQ_sub/Subsystem/EtherCATRobotMicrostrain/LegElmo_1R/Subsystem5 ==
  StatusWord : Inport
  Bitwise Operator : simulink/Logic and Bit Operations/Bitwise Operator  logicop=AND  UseBitMask=on  BitMask=bin2dec('0000000000001000')  BitMaskRealWorld=Stored Integer
  Compare To Constant : simulink/Logic and Bit Operations/Compare To Constant  relop===  const=bin2dec('0000000000001000')  OutDataTypeStr=boolean
  FaultMode : Outport
  wires:
  Bitwise Operator/1 -> Compare To Constant/1
  Compare To Constant/1 -> FaultMode/1
  StatusWord/1 -> Bitwise Operator/1

== system Controller_Exp/DAQ/DAQ_sub/Subsystem/EtherCATRobotMicrostrain/LegElmo_1R/Subsystem6 ==
  ScaledValue : Inport
  MaxRatedCurrent : Inport  Port=2
  Fcn : Fcn  Expr=u(1)*u(2)/1000
  Vector Concatenate : Concatenate
  ActualValue : Outport
  wires:
  Fcn/1 -> ActualValue/1
  MaxRatedCurrent/1 -> Vector Concatenate/2
  Vector Concatenate/1 -> Fcn/1
  ScaledValue/1 -> Vector Concatenate/1

== system Controller_Exp/DAQ/DAQ_sub/Subsystem/EtherCATRobotMicrostrain/LegElmo_2L/EtherCATSubsystem ==
  TargetTorque : Inport
  ControlWord : Inport  Port=2
  ModeOfOperation : Inport  Port=3
  EtherCAT PDO Receive : xpcethercatlib/EtherCAT PDO Receive  Priority=2  sig_name=Box 2 (Elmo Drive).Inputs.Torque actual value  sig_offset=2944  sig_type=int16  type_size=16  sig_dim=1  device_id=3  sample_time=0.001000
  EtherCAT PDO Receive1 : xpcethercatlib/EtherCAT PDO Receive  Priority=2  sig_name=Box 2 (Elmo Drive).Inputs.Position actual value  sig_offset=2912  sig_type=int32  type_size=32  sig_dim=1  device_id=3  sample_time=0.001000
  EtherCAT PDO Receive2 : xpcethercatlib/EtherCAT PDO Receive  Priority=2  sig_name=Box 2 (Elmo Drive).Inputs.Mode of operation display  sig_offset=2976  sig_type=int8  type_size=8  sig_dim=1  device_id=3  sample_time=0.001000
  EtherCAT PDO Receive5 : xpcethercatlib/EtherCAT PDO Receive  Priority=2  sig_name=Box 2 (Elmo Drive).Inputs.Status word  sig_offset=2960  sig_type=uint16  type_size=16  sig_dim=1  device_id=3  sample_time=0.001000
  EtherCAT PDO Transmit : xpcethercatlib/EtherCAT PDO Transmit   Priority=3  sig_name=Box 2 (Elmo Drive).Outputs.Target Torque  sig_offset=2912  sig_type=int16  type_size=16  sig_dim=1  device_id=3  sample_time=0.001000
  EtherCAT PDO Transmit1 : xpcethercatlib/EtherCAT PDO Transmit   Priority=3  sig_name=Box 2 (Elmo Drive).Outputs.Control word  sig_offset=2928  sig_type=uint16  type_size=16  sig_dim=1  device_id=3  sample_time=0.001000
  EtherCAT PDO Transmit2 : xpcethercatlib/EtherCAT PDO Transmit   Priority=3  sig_name=Box 2 (Elmo Drive).Outputs.Mode of operation  sig_offset=2944  sig_type=int8  type_size=8  sig_dim=1  device_id=3  sample_time=0.001000
  TorqueActual : Outport
  ActualPosition : Outport  Port=2
  ModeOfOperationDisplay : Outport  Port=3
  StatusWord : Outport  Port=4
  wires:
  EtherCAT PDO Receive5/1 -> StatusWord/1
  TargetTorque/1 -> EtherCAT PDO Transmit/1
  EtherCAT PDO Receive2/1 -> ModeOfOperationDisplay/1
  ModeOfOperation/1 -> EtherCAT PDO Transmit2/1
  ControlWord/1 -> EtherCAT PDO Transmit1/1
  EtherCAT PDO Receive1/1 -> ActualPosition/1
  EtherCAT PDO Receive/1 -> TorqueActual/1

== system Controller_Exp/DAQ/DAQ_sub/Subsystem/EtherCATRobotMicrostrain/LegElmo_2L/Subsystem ==
  ActualValue : Inport
  MaxRatedCurrent : Inport  Port=2
  Data Type Conversion6 : DataTypeConversion  OutDataTypeStr=int16
  Fcn : Fcn  Expr=u(1)*1000/u(2)
  Vector Concatenate : Concatenate
  ScaledValue : Outport
  wires:
  Fcn/1 -> Data Type Conversion6/1
  Data Type Conversion6/1 -> ScaledValue/1
  MaxRatedCurrent/1 -> Vector Concatenate/2
  Vector Concatenate/1 -> Fcn/1
  ActualValue/1 -> Vector Concatenate/1

== system Controller_Exp/DAQ/DAQ_sub/Subsystem/EtherCATRobotMicrostrain/LegElmo_2L/Subsystem1 ==
  ControlWordIndex : Inport
  EnableControlWord : Subsystem
  FaultReset : Subsystem
  Merge : Merge  Inputs=4
  NothingControlWord : Subsystem
  ShutdownControlWord : Subsystem
  Switch Case : SwitchCase  CaseConditions={1,2,3}
  ControlWord : Outport
  wires:
  FaultReset/1(ControlWord) -> Merge/3
  Switch Case/3 -> FaultReset/Action
  EnableControlWord/1(ControlWord) -> Merge/2
  ControlWordIndex/1 -> Switch Case/1
  Switch Case/2 -> EnableControlWord/Action
  Switch Case/4 -> NothingControlWord/Action
  ShutdownControlWord/1(ControlWord) -> Merge/1
  Switch Case/1 -> ShutdownControlWord/Action
  Merge/1 -> ControlWord/1
  NothingControlWord/1(ControlWord) -> Merge/4

== system Controller_Exp/DAQ/DAQ_sub/Subsystem/EtherCATRobotMicrostrain/LegElmo_2L/Subsystem2 ==
  StatusWord : Inport
  Bitwise Operator : simulink/Logic and Bit Operations/Bitwise Operator  logicop=AND  UseBitMask=on  BitMask=bin2dec('0000000001001111')  BitMaskRealWorld=Stored Integer
  Compare To Constant : simulink/Logic and Bit Operations/Compare To Constant  relop===  const=bin2dec('0000000001000000')  OutDataTypeStr=boolean
  SwitchOnDisabledMode : Outport
  wires:
  Bitwise Operator/1 -> Compare To Constant/1
  Compare To Constant/1 -> SwitchOnDisabledMode/1
  StatusWord/1 -> Bitwise Operator/1

== system Controller_Exp/DAQ/DAQ_sub/Subsystem/EtherCATRobotMicrostrain/LegElmo_2L/Subsystem3 ==
  StatusWord : Inport
  Bitwise Operator : simulink/Logic and Bit Operations/Bitwise Operator  logicop=AND  UseBitMask=on  BitMask=bin2dec('0000000001101111')  BitMaskRealWorld=Stored Integer
  Compare To Constant : simulink/Logic and Bit Operations/Compare To Constant  relop===  const=bin2dec('0000000000100111')  OutDataTypeStr=boolean
  EnabledMode : Outport
  wires:
  Bitwise Operator/1 -> Compare To Constant/1
  Compare To Constant/1 -> EnabledMode/1
  StatusWord/1 -> Bitwise Operator/1

== system Controller_Exp/DAQ/DAQ_sub/Subsystem/EtherCATRobotMicrostrain/LegElmo_2L/Subsystem4 ==
  StatusWord : Inport
  Bitwise Operator : simulink/Logic and Bit Operations/Bitwise Operator  logicop=AND  UseBitMask=on  BitMask=bin2dec('0000000001101111')  BitMaskRealWorld=Stored Integer
  Compare To Constant : simulink/Logic and Bit Operations/Compare To Constant  relop===  const=bin2dec('0000000000100001')  OutDataTypeStr=boolean
  ReadyToSwitchOnMode : Outport
  wires:
  Bitwise Operator/1 -> Compare To Constant/1
  Compare To Constant/1 -> ReadyToSwitchOnMode/1
  StatusWord/1 -> Bitwise Operator/1

== system Controller_Exp/DAQ/DAQ_sub/Subsystem/EtherCATRobotMicrostrain/LegElmo_2L/Subsystem5 ==
  StatusWord : Inport
  Bitwise Operator : simulink/Logic and Bit Operations/Bitwise Operator  logicop=AND  UseBitMask=on  BitMask=bin2dec('0000000000001000')  BitMaskRealWorld=Stored Integer
  Compare To Constant : simulink/Logic and Bit Operations/Compare To Constant  relop===  const=bin2dec('0000000000001000')  OutDataTypeStr=boolean
  FaultMode : Outport
  wires:
  Bitwise Operator/1 -> Compare To Constant/1
  Compare To Constant/1 -> FaultMode/1
  StatusWord/1 -> Bitwise Operator/1

== system Controller_Exp/DAQ/DAQ_sub/Subsystem/EtherCATRobotMicrostrain/LegElmo_2L/Subsystem6 ==
  ScaledValue : Inport
  MaxRatedCurrent : Inport  Port=2
  Fcn : Fcn  Expr=u(1)*u(2)/1000
  Vector Concatenate : Concatenate
  ActualValue : Outport
  wires:
  Fcn/1 -> ActualValue/1
  MaxRatedCurrent/1 -> Vector Concatenate/2
  Vector Concatenate/1 -> Fcn/1
  ScaledValue/1 -> Vector Concatenate/1

== system Controller_Exp/DAQ/DAQ_sub/Subsystem/EtherCATRobotMicrostrain/LegElmo_2R/EtherCATSubsystem ==
  TargetTorque : Inport
  ControlWord : Inport  Port=2
  ModeOfOperation : Inport  Port=3
  EtherCAT PDO Receive : xpcethercatlib/EtherCAT PDO Receive  Priority=2  sig_name=Box 9 (Elmo Drive).Inputs.Torque actual value  sig_offset=3104  sig_type=int16  type_size=16  sig_dim=1  device_id=3  sample_time=0.001000
  EtherCAT PDO Receive1 : xpcethercatlib/EtherCAT PDO Receive  Priority=2  sig_name=Box 9 (Elmo Drive).Inputs.Position actual value  sig_offset=3072  sig_type=int32  type_size=32  sig_dim=1  device_id=3  sample_time=0.001000
  EtherCAT PDO Receive3 : xpcethercatlib/EtherCAT PDO Receive  Priority=2  sig_name=Box 9 (Elmo Drive).Inputs.Mode of operation display  sig_offset=3136  sig_type=int8  type_size=8  sig_dim=1  device_id=3  sample_time=0.001000
  EtherCAT PDO Receive5 : xpcethercatlib/EtherCAT PDO Receive  Priority=2  sig_name=Box 9 (Elmo Drive).Inputs.Status word  sig_offset=3120  sig_type=uint16  type_size=16  sig_dim=1  device_id=3  sample_time=0.001000
  EtherCAT PDO Transmit : xpcethercatlib/EtherCAT PDO Transmit   Priority=3  sig_name=Box 9 (Elmo Drive).Outputs.Target Torque  sig_offset=3072  sig_type=int16  type_size=16  sig_dim=1  device_id=3  sample_time=0.001000
  EtherCAT PDO Transmit1 : xpcethercatlib/EtherCAT PDO Transmit   Priority=3  sig_name=Box 9 (Elmo Drive).Outputs.Control word  sig_offset=3088  sig_type=uint16  type_size=16  sig_dim=1  device_id=3  sample_time=0.001000
  EtherCAT PDO Transmit2 : xpcethercatlib/EtherCAT PDO Transmit   Priority=3  sig_name=Box 9 (Elmo Drive).Outputs.Mode of operation  sig_offset=3104  sig_type=int8  type_size=8  sig_dim=1  device_id=3  sample_time=0.001000
  TorqueActual : Outport
  ActualPosition : Outport  Port=2
  ModeOfOperationDisplay : Outport  Port=3
  StatusWord : Outport  Port=4
  wires:
  EtherCAT PDO Receive5/1 -> StatusWord/1
  TargetTorque/1 -> EtherCAT PDO Transmit/1
  ModeOfOperation/1 -> EtherCAT PDO Transmit2/1
  EtherCAT PDO Receive3/1 -> ModeOfOperationDisplay/1
  ControlWord/1 -> EtherCAT PDO Transmit1/1
  EtherCAT PDO Receive1/1 -> ActualPosition/1
  EtherCAT PDO Receive/1 -> TorqueActual/1

== system Controller_Exp/DAQ/DAQ_sub/Subsystem/EtherCATRobotMicrostrain/LegElmo_2R/Subsystem ==
  ActualValue : Inport
  MaxRatedCurrent : Inport  Port=2
  Data Type Conversion6 : DataTypeConversion  OutDataTypeStr=int16
  Fcn : Fcn  Expr=u(1)*1000/u(2)
  Vector Concatenate : Concatenate
  ScaledValue : Outport
  wires:
  Fcn/1 -> Data Type Conversion6/1
  Data Type Conversion6/1 -> ScaledValue/1
  MaxRatedCurrent/1 -> Vector Concatenate/2
  Vector Concatenate/1 -> Fcn/1
  ActualValue/1 -> Vector Concatenate/1

== system Controller_Exp/DAQ/DAQ_sub/Subsystem/EtherCATRobotMicrostrain/LegElmo_2R/Subsystem1 ==
  ControlWordIndex : Inport
  EnableControlWord : Subsystem
  FaultReset : Subsystem
  Merge : Merge  Inputs=4
  NothingControlWord : Subsystem
  ShutdownControlWord : Subsystem
  Switch Case : SwitchCase  CaseConditions={1,2,3}
  ControlWord : Outport
  wires:
  FaultReset/1(ControlWord) -> Merge/3
  Switch Case/3 -> FaultReset/Action
  EnableControlWord/1(ControlWord) -> Merge/2
  ControlWordIndex/1 -> Switch Case/1
  Switch Case/2 -> EnableControlWord/Action
  Switch Case/4 -> NothingControlWord/Action
  ShutdownControlWord/1(ControlWord) -> Merge/1
  Switch Case/1 -> ShutdownControlWord/Action
  Merge/1 -> ControlWord/1
  NothingControlWord/1(ControlWord) -> Merge/4

== system Controller_Exp/DAQ/DAQ_sub/Subsystem/EtherCATRobotMicrostrain/LegElmo_2R/Subsystem2 ==
  StatusWord : Inport
  Bitwise Operator : simulink/Logic and Bit Operations/Bitwise Operator  logicop=AND  UseBitMask=on  BitMask=bin2dec('0000000001001111')  BitMaskRealWorld=Stored Integer
  Compare To Constant : simulink/Logic and Bit Operations/Compare To Constant  relop===  const=bin2dec('0000000001000000')  OutDataTypeStr=boolean
  SwitchOnDisabledMode : Outport
  wires:
  Bitwise Operator/1 -> Compare To Constant/1
  Compare To Constant/1 -> SwitchOnDisabledMode/1
  StatusWord/1 -> Bitwise Operator/1

== system Controller_Exp/DAQ/DAQ_sub/Subsystem/EtherCATRobotMicrostrain/LegElmo_2R/Subsystem3 ==
  StatusWord : Inport
  Bitwise Operator : simulink/Logic and Bit Operations/Bitwise Operator  logicop=AND  UseBitMask=on  BitMask=bin2dec('0000000001101111')  BitMaskRealWorld=Stored Integer
  Compare To Constant : simulink/Logic and Bit Operations/Compare To Constant  relop===  const=bin2dec('0000000000100111')  OutDataTypeStr=boolean
  EnabledMode : Outport
  wires:
  Bitwise Operator/1 -> Compare To Constant/1
  Compare To Constant/1 -> EnabledMode/1
  StatusWord/1 -> Bitwise Operator/1

== system Controller_Exp/DAQ/DAQ_sub/Subsystem/EtherCATRobotMicrostrain/LegElmo_2R/Subsystem4 ==
  StatusWord : Inport
  Bitwise Operator : simulink/Logic and Bit Operations/Bitwise Operator  logicop=AND  UseBitMask=on  BitMask=bin2dec('0000000001101111')  BitMaskRealWorld=Stored Integer
  Compare To Constant : simulink/Logic and Bit Operations/Compare To Constant  relop===  const=bin2dec('0000000000100001')  OutDataTypeStr=boolean
  ReadyToSwitchOnMode : Outport
  wires:
  Bitwise Operator/1 -> Compare To Constant/1
  Compare To Constant/1 -> ReadyToSwitchOnMode/1
  StatusWord/1 -> Bitwise Operator/1

== system Controller_Exp/DAQ/DAQ_sub/Subsystem/EtherCATRobotMicrostrain/LegElmo_2R/Subsystem5 ==
  StatusWord : Inport
  Bitwise Operator : simulink/Logic and Bit Operations/Bitwise Operator  logicop=AND  UseBitMask=on  BitMask=bin2dec('0000000000001000')  BitMaskRealWorld=Stored Integer
  Compare To Constant : simulink/Logic and Bit Operations/Compare To Constant  relop===  const=bin2dec('0000000000001000')  OutDataTypeStr=boolean
  FaultMode : Outport
  wires:
  Bitwise Operator/1 -> Compare To Constant/1
  Compare To Constant/1 -> FaultMode/1
  StatusWord/1 -> Bitwise Operator/1

== system Controller_Exp/DAQ/DAQ_sub/Subsystem/EtherCATRobotMicrostrain/LegElmo_2R/Subsystem6 ==
  ScaledValue : Inport
  MaxRatedCurrent : Inport  Port=2
  Fcn : Fcn  Expr=u(1)*u(2)/1000
  Vector Concatenate : Concatenate
  ActualValue : Outport
  wires:
  Fcn/1 -> ActualValue/1
  MaxRatedCurrent/1 -> Vector Concatenate/2
  Vector Concatenate/1 -> Fcn/1
  ScaledValue/1 -> Vector Concatenate/1

== system Controller_Exp/DAQ/DAQ_sub/Subsystem/EncoderFilters/Filter/Velocity Filter/OSU_filter ==
  q : Inport
  Gain1 : Gain  Gain=1/sample_time
  difference : simulink/Discrete/Difference  ICPrevInput=0  InputProcessing=Columns as channels (frame based)  OutMin=[]  OutMax=[]  OutDataType=fixdt(1, 16)  OutScaling=2^-10  DoSatur=off
  two_pole_filter : DiscreteTransferFcn  Numerator=[A_lpf_velocity 0 0]  Denominator=[1 B1_lpf_velocity B2_lpf_velocity]  SampleTime=sample_time
  dq : Outport
  wires:
  difference/1 -> Gain1/1
  q/1 -> difference/1
  two_pole_filter/1 -> dq/1
  Gain1/1 -> two_pole_filter/1

== system Controller_Exp/DAQ/DAQ_sub/Subsystem/EncoderFilters1/CheckAndFilterEncoder/Velocity Filter/OSU_filter ==
  q : Inport
  Gain1 : Gain  Gain=1/sample_time
  difference : simulink/Discrete/Difference  ICPrevInput=0  InputProcessing=Columns as channels (frame based)  OutMin=[]  OutMax=[]  OutDataType=fixdt(1, 16)  OutScaling=2^-10  DoSatur=off
  two_pole_filter : DiscreteTransferFcn  Numerator=[A_lpf_velocity 0 0]  Denominator=[1 B1_lpf_velocity B2_lpf_velocity]  SampleTime=sample_time
  dq : Outport
  wires:
  difference/1 -> Gain1/1
  q/1 -> difference/1
  two_pole_filter/1 -> dq/1
  Gain1/1 -> two_pole_filter/1

== system Controller_Exp/DAQ/DAQ_sub/Subsystem/EtherCATRobotMicrostrain/LegElmo_1L/Subsystem1/EnableControlWord ==
  Action Port : ActionPort  ActionType=case
  Constant : Constant  Value=15  OutDataTypeStr=uint16
  ControlWord : Outport
  wires:
  Constant/1 -> ControlWord/1

== system Controller_Exp/DAQ/DAQ_sub/Subsystem/EtherCATRobotMicrostrain/LegElmo_1L/Subsystem1/FaultReset ==
  Action Port : ActionPort  ActionType=case
  Constant : Constant  Value=128  OutDataTypeStr=uint16
  ControlWord : Outport
  wires:
  Constant/1 -> ControlWord/1

== system Controller_Exp/DAQ/DAQ_sub/Subsystem/EtherCATRobotMicrostrain/LegElmo_1L/Subsystem1/NothingControlWord ==
  Action Port : ActionPort  ActionType=default
  Constant : Constant  Value=0  OutDataTypeStr=uint16
  ControlWord : Outport
  wires:
  Constant/1 -> ControlWord/1

== system Controller_Exp/DAQ/DAQ_sub/Subsystem/EtherCATRobotMicrostrain/LegElmo_1L/Subsystem1/ShutdownControlWord ==
  Action Port : ActionPort  ActionType=case
  Constant : Constant  Value=6  OutDataTypeStr=uint16
  ControlWord : Outport
  wires:
  Constant/1 -> ControlWord/1

== system Controller_Exp/DAQ/DAQ_sub/Subsystem/EtherCATRobotMicrostrain/LegElmo_1R/Subsystem1/EnableControlWord ==
  Action Port : ActionPort  ActionType=case
  Constant : Constant  Value=15  OutDataTypeStr=uint16
  ControlWord : Outport
  wires:
  Constant/1 -> ControlWord/1

== system Controller_Exp/DAQ/DAQ_sub/Subsystem/EtherCATRobotMicrostrain/LegElmo_1R/Subsystem1/FaultReset ==
  Action Port : ActionPort  ActionType=case
  Constant : Constant  Value=128  OutDataTypeStr=uint16
  ControlWord : Outport
  wires:
  Constant/1 -> ControlWord/1

== system Controller_Exp/DAQ/DAQ_sub/Subsystem/EtherCATRobotMicrostrain/LegElmo_1R/Subsystem1/NothingControlWord ==
  Action Port : ActionPort  ActionType=default
  Constant : Constant  Value=0  OutDataTypeStr=uint16
  ControlWord : Outport
  wires:
  Constant/1 -> ControlWord/1

== system Controller_Exp/DAQ/DAQ_sub/Subsystem/EtherCATRobotMicrostrain/LegElmo_1R/Subsystem1/ShutdownControlWord ==
  Action Port : ActionPort  ActionType=case
  Constant : Constant  Value=6  OutDataTypeStr=uint16
  ControlWord : Outport
  wires:
  Constant/1 -> ControlWord/1

== system Controller_Exp/DAQ/DAQ_sub/Subsystem/EtherCATRobotMicrostrain/LegElmo_2L/Subsystem1/EnableControlWord ==
  Action Port : ActionPort  ActionType=case
  Constant : Constant  Value=15  OutDataTypeStr=uint16
  ControlWord : Outport
  wires:
  Constant/1 -> ControlWord/1

== system Controller_Exp/DAQ/DAQ_sub/Subsystem/EtherCATRobotMicrostrain/LegElmo_2L/Subsystem1/FaultReset ==
  Action Port : ActionPort  ActionType=case
  Constant : Constant  Value=128  OutDataTypeStr=uint16
  ControlWord : Outport
  wires:
  Constant/1 -> ControlWord/1

== system Controller_Exp/DAQ/DAQ_sub/Subsystem/EtherCATRobotMicrostrain/LegElmo_2L/Subsystem1/NothingControlWord ==
  Action Port : ActionPort  ActionType=default
  Constant : Constant  Value=0  OutDataTypeStr=uint16
  ControlWord : Outport
  wires:
  Constant/1 -> ControlWord/1

== system Controller_Exp/DAQ/DAQ_sub/Subsystem/EtherCATRobotMicrostrain/LegElmo_2L/Subsystem1/ShutdownControlWord ==
  Action Port : ActionPort  ActionType=case
  Constant : Constant  Value=6  OutDataTypeStr=uint16
  ControlWord : Outport
  wires:
  Constant/1 -> ControlWord/1
